simulink model "penduldublu_liniarizat"  (R2022b)
settings: Solver=VariableStepAuto  StartTime=0.0  StopTime=45  RelTol=1e-3
values from neighbouring files (symbols this model uses):
  ustar = [0.1 ;0.5;0.82; 1;1.5; 1.8; 2 ; 2.8; 3.1;3.6;4;4.5;10]    [Main.m]
undefined symbols (not defined in the file or in its folder): A_lin, B_lin, C_lin, D_lin, xstar, ystar
settings Model: Creator=samue  LastModifiedBy=samue

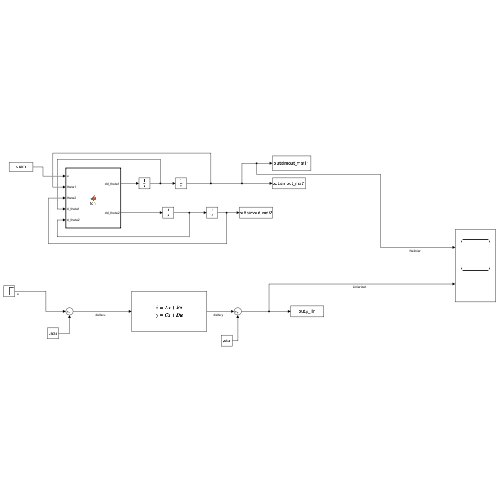
[thumbnail: Simulink's stored preview of the top-level diagram]
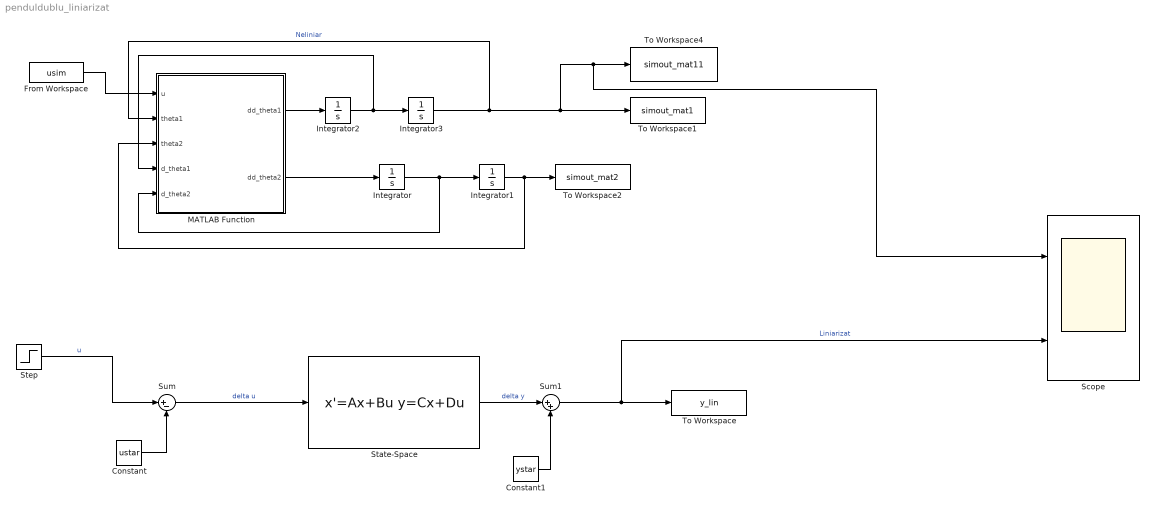
== system penduldublu_liniarizat ==
  Constant : Constant  Value=ustar
  Constant1 : Constant  Value=ystar
  From Workspace : FromWorkspace  VariableName=usim
  Integrator{,1..3} (4 alike) : Integrator
  MATLAB Function : MATLAB Function  TreatAsAtomicUnit=on
  Scope : Scope  NumInputPorts=2
  State-Space : StateSpace  A=A_lin  B=B_lin  C=C_lin  D=D_lin  InitialCondition=-xstar  AllowTunableDMatrix=on
  Step : Step  Time=0  After=1.5  SampleTime=0
  Sum : Sum  Inputs=|+-
  Sum1 : Sum  Inputs=|++
  To Workspace : ToWorkspace  VariableName=y_lin  SaveFormat=Timeseries  SampleTime=-1
  To Workspace1 : ToWorkspace  VariableName=simout_mat1  SampleTime=-1
      settings: Save2DSignal=2-D array (concatenate along first dimension)
  To Workspace2 : ToWorkspace  VariableName=simout_mat2  SampleTime=-1
      settings: Save2DSignal=2-D array (concatenate along first dimension)
  To Workspace4 : ToWorkspace  VariableName=simout_mat11  SaveFormat=Timeseries  SampleTime=-1
  wires:
  State-Space/1 -> Sum1/1  "delta y"
  Step/1 -> Sum/1  "u"
  Sum/1 -> State-Space/1  "delta u"
  Constant/1 -> Sum/2
  Constant1/1 -> Sum1/2
  Integrator2/1 -> MATLAB Function/4(d_theta1), Integrator3/1
  From Workspace/1 -> MATLAB Function/1(u)
  Integrator1/1 -> To Workspace2/1, MATLAB Function/3(theta2)
  Integrator/1 -> Integrator1/1, MATLAB Function/5(d_theta2)
  MATLAB Function/1(dd_theta1) -> Integrator2/1
  MATLAB Function/2(dd_theta2) -> Integrator/1
  Sum1/1 -> Scope/2, To Workspace/1  "Liniarizat"
  Integrator3/1 -> Scope/1, To Workspace4/1, To Workspace1/1, MATLAB Function/2(theta1)  "Neliniar"

== matlab function penduldublu_liniarizat/MATLAB Function ==
  data: u input; dd_theta1 output; theta1 input; theta2 input; d_theta1 input; d_theta2 input; dd_theta2 output
function [dd_theta1,dd_theta2] = fcn(u, theta1,theta2,d_theta1,d_theta2)
zeta = 0.7;
g = 10;
m = 5;
l = 1;

A = - (d_theta2^2) * sin(theta1 - theta2)   - 2 *g*sin(theta1)/l - zeta*d_theta1 + u/(m*l*l);
B =  (d_theta1^2 ) * sin(theta1 - theta2) - g*sin(theta2)/l - zeta*d_theta2;

dd_theta1 = (B* cos( theta1 - theta2)  - A )/( - cos(2*(theta1 - theta2)));
dd_theta2 = (2*B -A* cos( theta1 - theta2)    )/( cos(2*(theta1 - theta2)) );
